simulink model "NHR9200Model4904_2020b"  (R2020b)
settings: Solver=ode4  StartTime=0.0  StopTime=2  FixedStep=Ts  MaxStep=0.2  RelTol=1e-3
PreLoadFcn:
  | Ts=1e-3;
InitFcn:
  | Ts=1e-3;
libraries: simulink x31, fl_lib x15, nesl_utility x14, simulink_extras x6, powerlib_meascontrol x6, ee_lib x2
(part 2 of 2)

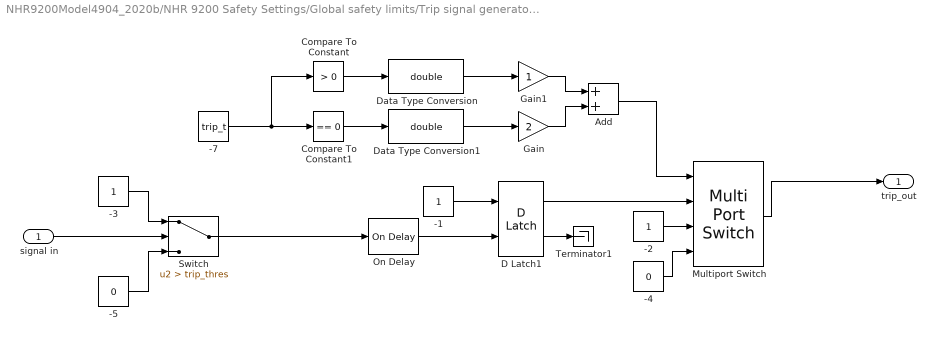
== system NHR9200Model4904_2020b/NHR 9200 Safety Settings/Global safety limits/Trip signal generator (max) Voltage/trip signal gen ==
  signal in : Inport
  -1 : Constant  OutDataTypeStr=boolean
  -2 : Constant  OutDataTypeStr=boolean
  -3 : Constant  OutDataTypeStr=boolean
  -4 : Constant  Value=0  OutDataTypeStr=boolean
  -5 : Constant  Value=0  OutDataTypeStr=boolean
  -7 : Constant  Value=trip_t  OutDataTypeStr=boolean
  Add : Sum
  Compare To Constant : simulink/Logic and Bit Operations/Compare To Constant  relop=>  const=0  OutDataTypeStr=uint8
  Compare To Constant1 : simulink/Logic and Bit Operations/Compare To Constant  relop===  const=0  OutDataTypeStr=uint8
  D Latch1 : simulink_extras/Flip Flops/D Latch
      settings: SourceProductBaseCode=SL
  Data Type Conversion : DataTypeConversion  OutDataTypeStr=double
  Data Type Conversion1 : DataTypeConversion  OutDataTypeStr=double
  Gain : Gain  Gain=2
  Gain1 : Gain
  Multiport Switch : MultiPortSwitch  Inputs=2  DataPortForDefault=Additional data port
  On Delay : powerlib_meascontrol/Logic/On Delay  DelayType=On delay  delay=trip_t  ic=0  Ts=0
  Switch : Switch  Criteria=u2 > Threshold  Threshold=trip_thres
  Terminator1 : Terminator
  trip_out : Outport  VectorParamsAs1DForOutWhenUnconnected=off
  wires:
  Switch/1 -> On Delay/1
  On Delay/1 -> D Latch1/2
  D Latch1/1 -> Multiport Switch/2
  -4/1 -> Multiport Switch/4
  Multiport Switch/1 -> trip_out/1
  -2/1 -> Multiport Switch/3
  -3/1 -> Switch/1
  -5/1 -> Switch/3
  D Latch1/2 -> Terminator1/1
  signal in/1 -> Switch/2
  -7/1 -> Compare To Constant1/1, Compare To Constant/1
  Gain1/1 -> Add/1
  Gain/1 -> Add/2
  Data Type Conversion1/1 -> Gain/1
  Compare To Constant1/1 -> Data Type Conversion1/1
  Add/1 -> Multiport Switch/1
  Data Type Conversion/1 -> Gain1/1
  Compare To Constant/1 -> Data Type Conversion/1
  -1/1 -> D Latch1/1

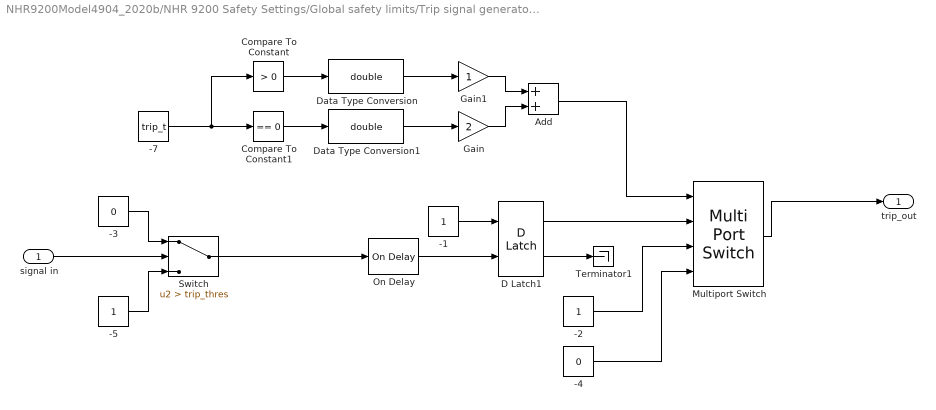
== system NHR9200Model4904_2020b/NHR 9200 Safety Settings/Global safety limits/Trip signal generator (min) Voltage/trip signal gen ==
  signal in : Inport
  -1 : Constant  OutDataTypeStr=boolean
  -2 : Constant  OutDataTypeStr=boolean
  -3 : Constant  Value=0  OutDataTypeStr=boolean
  -4 : Constant  Value=0  OutDataTypeStr=boolean
  -5 : Constant  OutDataTypeStr=boolean
  -7 : Constant  Value=trip_t  OutDataTypeStr=boolean
  Add : Sum
  Compare To Constant : simulink/Logic and Bit Operations/Compare To Constant  relop=>  const=0  OutDataTypeStr=uint8
  Compare To Constant1 : simulink/Logic and Bit Operations/Compare To Constant  relop===  const=0  OutDataTypeStr=uint8
  D Latch1 : simulink_extras/Flip Flops/D Latch
      settings: SourceProductBaseCode=SL
  Data Type Conversion : DataTypeConversion  OutDataTypeStr=double
  Data Type Conversion1 : DataTypeConversion  OutDataTypeStr=double
  Gain : Gain  Gain=2
  Gain1 : Gain
  Multiport Switch : MultiPortSwitch  Inputs=2  DataPortForDefault=Additional data port
  On Delay : powerlib_meascontrol/Logic/On Delay  DelayType=On delay  delay=trip_t  ic=0  Ts=0
  Switch : Switch  Criteria=u2 > Threshold  Threshold=trip_thres
  Terminator1 : Terminator
  trip_out : Outport  VectorParamsAs1DForOutWhenUnconnected=off
  wires:
  signal in/1 -> Switch/2
  D Latch1/2 -> Terminator1/1
  -1/1 -> D Latch1/1
  -5/1 -> Switch/3
  -3/1 -> Switch/1
  -2/1 -> Multiport Switch/3
  Multiport Switch/1 -> trip_out/1
  -4/1 -> Multiport Switch/4
  D Latch1/1 -> Multiport Switch/2
  On Delay/1 -> D Latch1/2
  Switch/1 -> On Delay/1
  Gain1/1 -> Add/1
  Compare To Constant/1 -> Data Type Conversion/1
  Gain/1 -> Add/2
  Compare To Constant1/1 -> Data Type Conversion1/1
  Data Type Conversion1/1 -> Gain/1
  -7/1 -> Compare To Constant1/1, Compare To Constant/1
  Data Type Conversion/1 -> Gain1/1
  Add/1 -> Multiport Switch/1

== matlab function NHR9200Model4904_2020b/NHR 9200/NHR 9200 Discharging mode1/sink_control/MATLAB Function1 ==
  data: p input; i input; y output; x input
function y = fcn(p,i,x)
tol=1e-3;
gain=1e-4;
Ts=1e-3;
if p<=(-tol)
    y=x-(gain/Ts);
elseif i<=(-tol)
    y=x-(gain/Ts);
elseif i>tol;
    y=x+(gain/Ts);
else
    y=0;
end

== matlab function NHR9200Model4904_2020b/NHR 9200/NHR 9200 Charging mode/source_control/MATLAB Function ==
  data: p input; v input; y output; i input; x input
function y = fcn(p,v,i,x)
tol=1e-3;
gain=1e-4;
Ts=1e-3;
if p<=(-tol)
    y=x-(gain/Ts);
elseif i<=(-tol)
    y=x-(gain/Ts);
elseif v<=(-tol)
    y=x-(gain/Ts);
elseif v>tol;
    y=x+(gain/Ts);
else
    y=0;
end
